simulink model "DrivetrainAndMotor"  (R2015a)
settings: Solver=ode45  StartTime=0.0  StopTime=5  RelTol=1e-3
values from neighbouring files (symbols this model uses):
  Btot = 4.7088e-6    (= 4.7088e-06)    [motormodelscriptsimulink.m]
  Jtot = 5.5980e-06    (= 5.598e-06)    [motormodelscriptsimulink.m]
  Ke = 1.89e-3    (= 0.00189)    [motormodelscriptsimulink.m]
  Kt = 0.0016    [motormodelscriptsimulink.m]
  L = 119.26e-6    (= 0.00011926)    [motormodelscriptsimulink.m]
  N = 187/4773    (= 0.0391787135973)    [motormodelscriptsimulink.m]
  R = 0.178    [motormodelscriptsimulink.m]
  rt = 0.166/(2*pi)    (= 0.0264197205533)    [motormodelscriptsimulink.m]
libraries: simulink x2
settings Model: Creator=Amalie  LastModifiedBy=Amalie

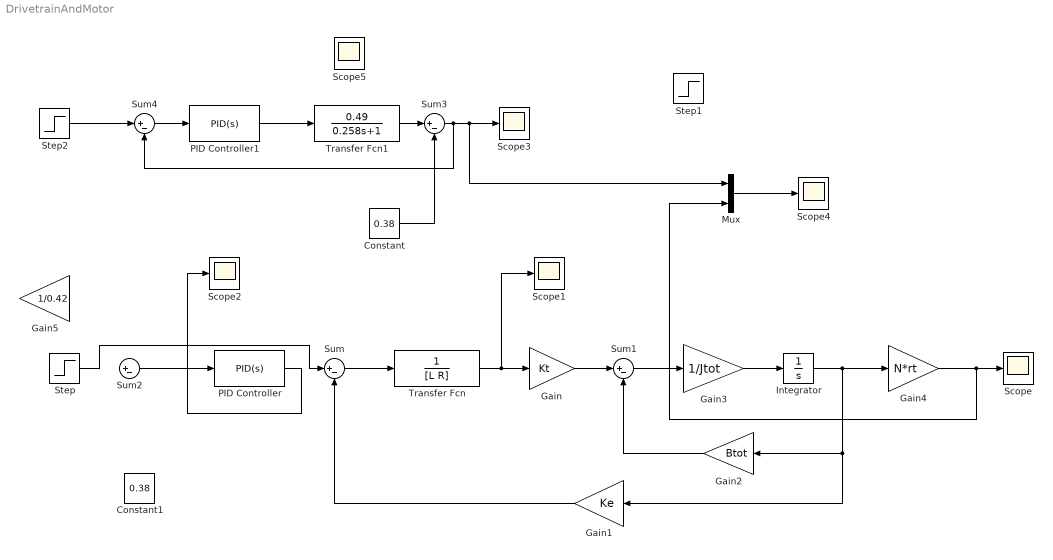
== system DrivetrainAndMotor ==
  Constant : Constant  Value=0.38
  Constant1 : Constant  Value=0.38
  Gain : Gain  Gain=Kt
  Gain1 : Gain  Gain=Ke
  Gain2 : Gain  Gain=Btot
  Gain3 : Gain  Gain=1/Jtot
  Gain4 : Gain  Gain=N*rt
  Gain5 : Gain  Gain=1/0.42
  Integrator : Integrator
  Mux : Mux  Inputs=2
  PID Controller : simulink/Continuous/PID Controller  Controller=PID  TimeDomain=Continuous-time  SampleTime=-1  IntegratorMethod=Forward Euler  FilterMethod=Forward Euler  Form=Parallel  UseFilter=on  ControllerParametersSource=internal  P=10  I=0  D=0  N=0  InitialConditionSource=internal  InitialConditionForIntegrator=0  InitialConditionForFilter=0  ExternalReset=none  LimitOutput=on  UpperSaturationLimit=6.83  LowerSaturationLimit=0  LinearizeAsGain=on  AntiWindupMode=none  Kb=1  TrackingMode=off  Kt=1  PParamMin=[]  PParamMax=[]  IParamMin=[]  IParamMax=[]  DParamMin=[]  DParamMax=[]  NParamMin=[]  NParamMax=[]  KbParamMin=[]  KbParamMax=[]  KtParamMin=[]  KtParamMax=[]  POutMin=[]  POutMax=[]  IOutMin=[]  IOutMax=[]  DOutMin=[]  DOutMax=[]  NOutMin=[]  NOutMax=[]  KbOutMin=[]  KbOutMax=[]  KtOutMin=[]  KtOutMax=[]  IntegratorOutMin=[]  IntegratorOutMax=[]  FilterOutMin=[]  FilterOutMax=[]  SumOutMin=[]  SumOutMax=[]  SumI1OutMin=[]  SumI1OutMax=[]  SumI2OutMin=[]  SumI2OutMax=[]  SumI3OutMin=[]  SumI3OutMax=[]  SumDOutMin=[]  SumDOutMax=[]  SaturationOutMin=[]  SaturationOutMax=[]  IntegratorContinuousStateAttributes=''  IntegratorStateMustResolveToSignalObject=off  IntegratorRTWStateStorageClass=Auto  FilterContinuousStateAttributes=''  FilterStateMustResolveToSignalObject=off  FilterRTWStateStorageClass=Auto  DifferentiatorICPrevScaledInput=0  DifferentiatorOutMin=[]  DifferentiatorOutMax=[]
  PID Controller1 : simulink/Continuous/PID Controller  Controller=PID  TimeDomain=Continuous-time  SampleTime=-1  IntegratorMethod=Forward Euler  FilterMethod=Forward Euler  Form=Parallel  UseFilter=on  ControllerParametersSource=internal  P=1  I=0  D=0  N=0  InitialConditionSource=internal  InitialConditionForIntegrator=0  InitialConditionForFilter=0  ExternalReset=none  LimitOutput=on  UpperSaturationLimit=6.83  LowerSaturationLimit=0  LinearizeAsGain=on  AntiWindupMode=none  Kb=1  TrackingMode=off  Kt=1  PParamMin=[]  PParamMax=[]  IParamMin=[]  IParamMax=[]  DParamMin=[]  DParamMax=[]  NParamMin=[]  NParamMax=[]  KbParamMin=[]  KbParamMax=[]  KtParamMin=[]  KtParamMax=[]  POutMin=[]  POutMax=[]  IOutMin=[]  IOutMax=[]  DOutMin=[]  DOutMax=[]  NOutMin=[]  NOutMax=[]  KbOutMin=[]  KbOutMax=[]  KtOutMin=[]  KtOutMax=[]  IntegratorOutMin=[]  IntegratorOutMax=[]  FilterOutMin=[]  FilterOutMax=[]  SumOutMin=[]  SumOutMax=[]  SumI1OutMin=[]  SumI1OutMax=[]  SumI2OutMin=[]  SumI2OutMax=[]  SumI3OutMin=[]  SumI3OutMax=[]  SumDOutMin=[]  SumDOutMax=[]  SaturationOutMin=[]  SaturationOutMax=[]  IntegratorContinuousStateAttributes=''  IntegratorStateMustResolveToSignalObject=off  IntegratorRTWStateStorageClass=Auto  FilterContinuousStateAttributes=''  FilterStateMustResolveToSignalObject=off  FilterRTWStateStorageClass=Auto  DifferentiatorICPrevScaledInput=0  DifferentiatorOutMin=[]  DifferentiatorOutMax=[]
  Scope{,1..5} (6 alike) : Scope
      Scope settings: TimeRange=10
      Scope2 settings: SaveName=ScopeData2
      Scope3 settings: TimeRange=10  SaveName=ScopeData3
      Scope4 settings: TimeRange=10  SaveName=ScopeData4
      Scope5 settings: SaveName=ScopeData5
  Step : Step  After=7  SampleTime=0
  Step1 : Step  Time=1.0  Before=0.7  After=7  SampleTime=0
  Step2 : Step  Time=1.0  After=7  SampleTime=0
  Sum{,1..4} (5 alike) : Sum  Inputs=|+-
  Transfer Fcn : TransferFcn  Denominator=[L R]
  Transfer Fcn1 : TransferFcn  Numerator=[0.49]  Denominator=[0.258 1]
  wires:
  Transfer Fcn/1 -> Scope1/1, Gain/1
  Gain1/1 -> Sum/2
  Gain2/1 -> Sum1/2
  Sum1/1 -> Gain3/1
  Gain3/1 -> Integrator/1
  Gain/1 -> Sum1/1
  Sum/1 -> Transfer Fcn/1
  Sum2/1 -> PID Controller/1
  Integrator/1 -> Gain4/1, Gain1/1, Gain2/1
  Gain4/1 -> Mux/2, Scope/1
  PID Controller/1 -> Scope2/1
  Mux/1 -> Scope4/1
  Transfer Fcn1/1 -> Sum3/1
  Constant/1 -> Sum3/2
  Sum3/1 -> Sum4/2, Mux/1, Scope3/1
  Step/1 -> Sum/1
  Step2/1 -> Sum4/1
  Sum4/1 -> PID Controller1/1
  PID Controller1/1 -> Transfer Fcn1/1
